simulink model "w1project1"  (R2020b)
settings: Solver=VariableStepAuto  StartTime=0.0  StopTime=inf  RelTol=1e-3
settings Model: PacingRate=1.100000  Creator=rutvi  LastModifiedBy=rutvi

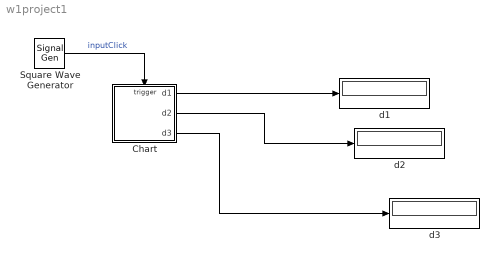
== system w1project1 ==
  Chart : Stateflow chart  TreatAsAtomicUnit=on
  Square Wave Generator : SignalGenerator  WaveForm=square  Units=rad/sec
  d1 : Display
  d2 : Display
  d3 : Display
  wires:
  Square Wave Generator/1 -> Chart/Trigger  "inputClick"
  Chart/1(d1) -> d1/1
  Chart/2(d2) -> d2/1
  Chart/3(d3) -> d3/1

== stateflow chart w1project1/Chart ==
  state digit3 [parallel]
    settings: executionOrder=3
    state one
      en: d3 = 1;
    state two
      en: d3 = 2;
    state zero
      en: d3 = 0;
    state four
      en:d3=4;
    state three
      en:d3=3;
    digit3.zero -> digit3.one : inc3
    digit3.one -> digit3.two : inc3
    (default) -> digit3.zero
    digit3.four -> digit3.zero : inc3
    digit3.two -> digit3.three : inc3
    digit3.three -> digit3.four : inc3
  state digit2 [parallel]
    settings: executionOrder=2
    state one
      en: d2 = 1;
    state two
      en: d2 = 2;
    state zero
      en: d2 = 0;
    state four
      en:d2=4;
    state three
      en:d2=3;
    digit2.zero -> digit2.one : inc2
    digit2.one -> digit2.two : inc2
    (default) -> digit2.zero
    digit2.four -> digit2.zero : inc2{digit3.inc3;}
    digit2.two -> digit2.three : inc2
    digit2.three -> digit2.four : inc2
  state digit1 [parallel]
    settings: executionOrder=1
    state one
      en: d1 = 1;
    state two
      en: d1 = 2;
    state zero
      en: d1 = 0;
    state three
      en:d1=3;
    state four
      en:d1=4;
    digit1.zero -> digit1.one : inputClick
    digit1.one -> digit1.two : inputClick
    (default) -> digit1.zero
    digit1.four -> digit1.zero : inputClick{digit2.inc2;}
    digit1.two -> digit1.three : inputClick
    digit1.three -> digit1.four : inputClick
  data: d1 output; d2 output; d3 output
  events: inc3 local FUNCTION_CALL_EVENT; inc2 local FUNCTION_CALL_EVENT; inputClick input EITHER_EDGE_EVENT
